simulink model "ThreePhasePWMSplitInverter"  (R2024b)
settings: Solver=FixedStepAuto  StartTime=0.0  StopTime=.1  FixedStep=1e-6  RelTol=1e-3
PreLoadFcn:
  | run('D:\Mtech_IIT_DH\Academics\S2\Subjects\Power Electronics\Simulink Projects and homework\Assignment 1 Three phase Inverter PWM\parameter.m');
values from neighbouring files (symbols this model uses):
  Fsig = 314.16    [parameter.m]
  L = 0.08    [parameter.m]
  Rl = 80    [parameter.m]
  Vdc = 200    [parameter.m]
libraries: spsMosfetLib x6, spsDCVoltageSourceLib x2, spsGroundLib x2, spsThreePhaseSeriesRLCBranchLib x2, spsThreePhaseVIMeasurementLib x2, spsSawtoothGeneratorLib x1, sps_lib x1
settings Model: Creator=Yadu  LastModifiedBy=Yadu

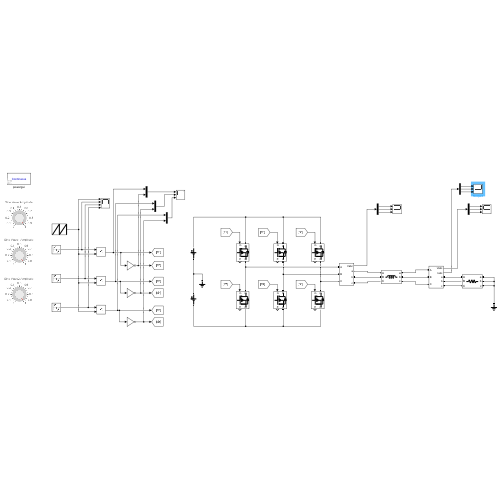
[thumbnail: Simulink's stored preview of the top-level diagram]
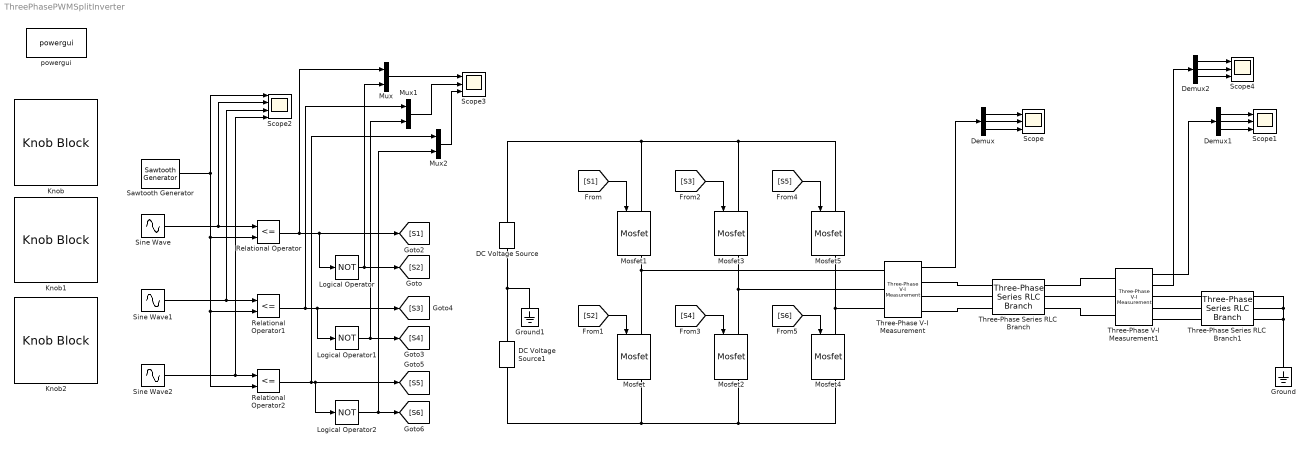
== system ThreePhasePWMSplitInverter ==
  DC Voltage Source : spsDCVoltageSourceLib/DC Voltage Source  Amplitude=Vdc  Measurements=None
  DC Voltage Source1 : spsDCVoltageSourceLib/DC Voltage Source  Amplitude=Vdc  Measurements=None
  Demux : Demux  Outputs=3
  Demux1 : Demux  Outputs=3
  Demux2 : Demux  Outputs=3
  Ground : spsGroundLib/Ground  LConnTagsString=a
  Ground1 : spsGroundLib/Ground  LConnTagsString=a
  Knob : KnobBlock  ScaleMax=1  TickInterval=.1
  Knob1 : KnobBlock  ScaleMax=1  TickInterval=.1
  Knob2 : KnobBlock  ScaleMax=1  TickInterval=.1
  Logical Operator : Logic  Operator=NOT  IconShape=distinctive  AllPortsSameDT=off  OutDataTypeStr=boolean
  Logical Operator1 : Logic  Operator=NOT  IconShape=distinctive  AllPortsSameDT=off  OutDataTypeStr=boolean
  Logical Operator2 : Logic  Operator=NOT  IconShape=distinctive  AllPortsSameDT=off  OutDataTypeStr=boolean
  Mosfet{,1..5} (6 alike) : spsMosfetLib/Mosfet  Ron=0.1  Lon=0  Rd=0.01  Vfd=0  IC=0  Rs=1e5  Cs=inf  Measurements=on
  Mux : Mux  Inputs=2
  Mux1 : Mux  Inputs=2
  Mux2 : Mux  Inputs=2
  Relational Operator : RelationalOperator  Operator=<=  OutDataTypeStr=boolean  RndMeth=Simplest  InputSameDT=off
  Relational Operator1 : RelationalOperator  Operator=<=  OutDataTypeStr=boolean  RndMeth=Simplest  InputSameDT=off
  Relational Operator2 : RelationalOperator  Operator=<=  OutDataTypeStr=boolean  RndMeth=Simplest  InputSameDT=off
  Sawtooth Generator : spsSawtoothGeneratorLib/Sawtooth Generator  Freq=Fs  Phase=0  Ts=0
  Scope{,1,3..4} (4 alike) : Scope  NumInputPorts=3
  Scope2 : Scope  NumInputPorts=4
  Sine Wave : Sin  Frequency=Fsig  SampleTime=0
  Sine Wave1 : Sin  Frequency=Fsig  Phase=2*pi/3  SampleTime=0
  Sine Wave2 : Sin  Frequency=Fsig  Phase=-2*pi/3  SampleTime=0
  Three-Phase Series RLC Branch : spsThreePhaseSeriesRLCBranchLib/Three-Phase Series RLC Branch  LConnTagsString=A|B|C  RConnTagsString=A|B|C  BranchType=L  Resistance=10  Inductance=L  Capacitance=0  Measurements=None
  Three-Phase Series RLC Branch1 : spsThreePhaseSeriesRLCBranchLib/Three-Phase Series RLC Branch  LConnTagsString=A|B|C  RConnTagsString=A|B|C  BranchType=R  Resistance=Rl  Inductance=1e-3  Capacitance=1e-6  Measurements=None
  Three-Phase V-I Measurement : spsThreePhaseVIMeasurementLib/Three-Phase V-I Measurement  VoltageMeasurement=phase-to-ground  SetLabelV=off  LabelV=Vabc  Vpu=off  VpuLL=off  CurrentMeasurement=no  SetLabelI=off  LabelI=Iabc  Ipu=off  Pbase=100e6  Vbase=500e3  OutputType=Complex  PhasorSimulation=off  PSBequivalent=0
  Three-Phase V-I Measurement1 : spsThreePhaseVIMeasurementLib/Three-Phase V-I Measurement  VoltageMeasurement=phase-to-ground  SetLabelV=off  LabelV=Vabc  Vpu=off  VpuLL=off  CurrentMeasurement=yes  SetLabelI=off  LabelI=Iabc  Ipu=off  Pbase=100e6  Vbase=500e3  OutputType=Complex  PhasorSimulation=off  PSBequivalent=0
  powergui : sps_lib/powergui  Priority=1  SimulationMode=Continuous  SampleTime=50e-6  frequency=60  Iterations=50  frequencyindice=0  Pbase=100e6  ErrMax=1e-4  UnitsV=kV  UnitsW=MW  buscounter=0  FunctionMessages=off  echomessages=off  EnableUseOfTLC=off  CurrentSourceSwitches=off  DisableSnubberDevices=off  DisableRonSwitches=off  DisableVfSwitches=off  DisplayEquations=off  AutomaticDiscreteSolvers=off  SolverType=Tustin/Backward Euler (TBE)  Interpol=off  ExternalGateDelay=off  methode=off  Ts=100  x0status=blocks  SPID=on  SwTol=0  HookPort=off  NonlinearTolerance=1e-4  nMaxIteration=100  ContinueOnMaxIteration=off  RestoreLinks=warning  ResistiveCurrentMeasurement=off  Frange=[0:2:500]  Ylog=off  Xlog=on  ShowGrid=off  save=off  variable=ZData  structure=0  ZoomFFT=off  StartTime=0.0  cycles=1  DisplayStyle=1  fundamental=60  FreqAxis=off  MaxFrequency=1000  frequencyindicesteady=1  RmsSteady=1  display=off
  wires:
  Demux/1 -> Scope/1
  Demux/2 -> Scope/2
  Demux/3 -> Scope/3
  Demux1/1 -> Scope1/1
  Demux1/2 -> Scope1/2
  Demux1/3 -> Scope1/3
  Three-Phase V-I Measurement/1 -> Demux/1
  Three-Phase V-I Measurement1/1 -> Demux1/1
  [S1] -> Mosfet1/1
  [S2] -> Mosfet/1
  [S4] -> Mosfet2/1
  [S3] -> Mosfet3/1
  [S5] -> Mosfet5/1
  [S6] -> Mosfet4/1
  Logical Operator/1 -> Mux/2, [S2]
  Relational Operator1/1 -> Mux1/1, Logical Operator1/1, [S3]
  Logical Operator1/1 -> Mux1/2, [S4]
  Relational Operator/1 -> Mux/1, Logical Operator/1, [S1]
  Relational Operator2/1 -> [S5], Logical Operator2/1, Mux2/1
  Logical Operator2/1 -> Mux2/2, [S6]
  Sine Wave/1 -> Scope2/2, Relational Operator/1
  Sine Wave1/1 -> Scope2/3, Relational Operator1/1
  Sine Wave2/1 -> Scope2/4, Relational Operator2/1
  Sawtooth Generator/1 -> Scope2/1, Relational Operator2/2, Relational Operator1/2, Relational Operator/2
  Mux1/1 -> Scope3/2
  Mux/1 -> Scope3/1
  Mux2/1 -> Scope3/3
  Demux2/3 -> Scope4/3
  Demux2/2 -> Scope4/2
  Demux2/1 -> Scope4/1
  Three-Phase V-I Measurement1/2 -> Demux2/1
  connections:
  Three-Phase V-I Measurement/RConn1 -- Three-Phase Series RLC Branch/LConn1
  Three-Phase V-I Measurement/RConn2 -- Three-Phase Series RLC Branch/LConn2
  Three-Phase V-I Measurement/RConn3 -- Three-Phase Series RLC Branch/LConn3
  Mosfet1/RConn1 -- Three-Phase V-I Measurement/LConn1 -- Mosfet/LConn1
  Mosfet3/RConn1 -- Three-Phase V-I Measurement/LConn2 -- Mosfet2/LConn1
  Mosfet5/RConn1 -- Three-Phase V-I Measurement/LConn3 -- Mosfet4/LConn1
  DC Voltage Source/LConn1 -- Ground1/LConn1 -- DC Voltage Source1/RConn1
  DC Voltage Source1/LConn1 -- Mosfet/RConn1 -- Mosfet2/RConn1 -- Mosfet4/RConn1
  DC Voltage Source/RConn1 -- Mosfet1/LConn1 -- Mosfet3/LConn1 -- Mosfet5/LConn1
  Three-Phase V-I Measurement1/LConn1 -- Three-Phase Series RLC Branch/RConn1
  Three-Phase V-I Measurement1/LConn2 -- Three-Phase Series RLC Branch/RConn2
  Three-Phase V-I Measurement1/LConn3 -- Three-Phase Series RLC Branch/RConn3
  Three-Phase Series RLC Branch1/RConn1 -- Three-Phase Series RLC Branch1/RConn2 -- Three-Phase Series RLC Branch1/RConn3 -- Ground/LConn1
  Three-Phase V-I Measurement1/RConn1 -- Three-Phase Series RLC Branch1/LConn1
  Three-Phase V-I Measurement1/RConn2 -- Three-Phase Series RLC Branch1/LConn2
  Three-Phase V-I Measurement1/RConn3 -- Three-Phase Series RLC Branch1/LConn3
